simulink model "sim_WAM_PBRCDynamics"  (R2018b)
settings: Solver=FixedStepAuto  StartTime=0.0  StopTime=2  FixedStep=1e-3  RelTol=1e-3
values from neighbouring files (symbols this model uses):
  Cfcn = matlabFunction(Ctemp, 'vars', {q1, q2, q4, q1d, q2d, q4d})    [convertSymVarsTOfunctions.m]
  Ffcn = matlabFunction(Ftemp, 'vars', {q1d, q2d, q4d})    [convertSymVarsTOfunctions.m]
  Gfcn = matlabFunction(Gtemp, 'vars', {q1, q2, q4})    [convertSymVarsTOfunctions.m]
  handles =     [opt.mat]
  K = diag([10 30 10])    [MAIN_FINAL.m]    (also in PBMC_WAM.m = 10*diag([1 1 1]))
  Lambda = 5*eye(3)    [MAIN_FINAL.m]    (also in PBMC_WAM.m = 10*diag([1 1 1]))
  Mfcn = matlabFunction(Mtemp, 'vars', {q1, q2, q4})    [convertSymVarsTOfunctions.m]
  rho = 10    [MAIN_FINAL.m]
  TH0 = TH    [MAIN_FINAL.m]
  w = 2*pi/10    (= 0.628318530718)    [GetOptimalTrajectories.m]    (also in MAIN_FINAL.m = 1; MAIN_OptimalTrajectories.m; invDynWAM.m = 4; trajct1.mat)
  Yavfcn = matlabFunction(Yavtemp, 'vars', {q1, q2, q4, q1d, q2d, q4d, q1dd, q2dd, q4dd,                                                  v1, v2, v3, a1, a2, a3})    [convertSymVarsTOfunctions.m]
undefined symbols (not defined in the file or in its folder): getOptimal, PBRC_WAM, statederWAM
settings Model: Creator=Erivelton  LastModifiedBy=Erivelton

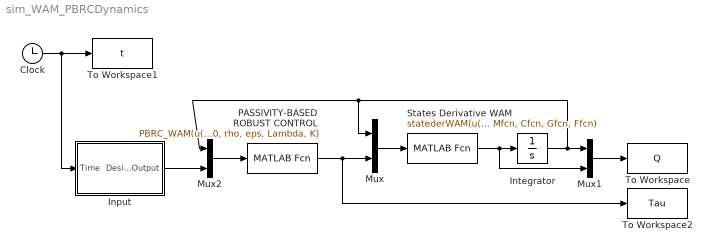
== system sim_WAM_PBRCDynamics ==
  Clock : Clock
  Input : Subsystem
  Integrator : Integrator  InitialCondition=handles.Q0
  Mux : Mux  Inputs=2
  Mux1 : Mux  Inputs=2
  Mux2 : Mux  Inputs=2
  PASSIVITY-BASED ROBUST CONTROL : MATLABFcn  MATLABFcn=PBRC_WAM(u(1:6), u(7:15), Yavfcn, TH0, rho, eps, Lambda, K)  OutputDimensions=3
  States Derivative WAM : MATLABFcn  MATLABFcn=statederWAM(u(1:6), u(7:9), Mfcn, Cfcn, Gfcn, Ffcn)  OutputDimensions=6
  To Workspace : ToWorkspace  VariableName=Q  SampleTime=-1
  To Workspace1 : ToWorkspace  VariableName=t  SampleTime=-1
  To Workspace2 : ToWorkspace  VariableName=Tau  SampleTime=-1
  wires:
  States Derivative WAM/1 -> Mux1/2, Integrator/1
  Mux/1 -> States Derivative WAM/1
  Integrator/1 -> Mux1/1, Mux/1, Mux2/1
  Clock/1 -> Input/1("Time "), To Workspace1/1
  Mux1/1 -> To Workspace/1
  PASSIVITY-BASED ROBUST CONTROL/1 -> To Workspace2/1, Mux/2
  Input/1(Desired Output) -> Mux2/2
  Mux2/1 -> PASSIVITY-BASED ROBUST CONTROL/1

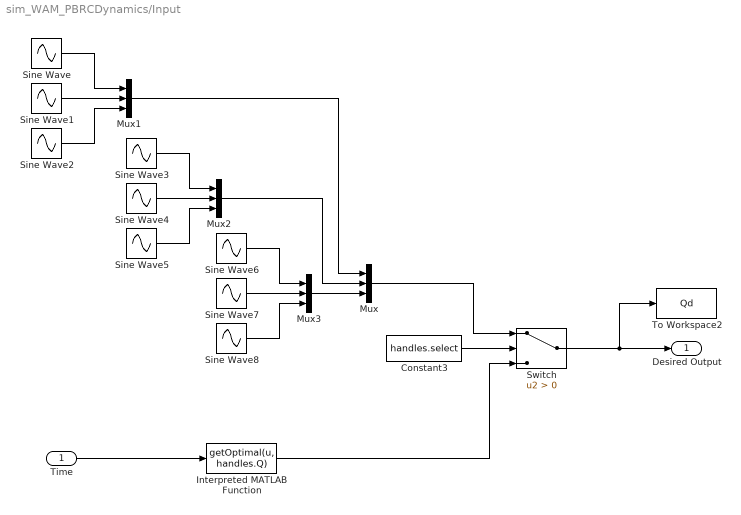
== system sim_WAM_PBRCDynamics/Input ==
  "Time " : Inport
  Constant3 : Constant  Value=handles.select
  Interpreted MATLAB Function : MATLABFcn  MATLABFcn=getOptimal(u, handles.Q)
  Mux{,1..3} (4 alike) : Mux  Inputs=3
  Sine Wave : Sin  Frequency=w  SampleTime=0
  Sine Wave1 : Sin  Amplitude=w  Frequency=w  Phase=pi/2  SampleTime=0
  Sine Wave2 : Sin  Amplitude=-w*w  Frequency=w  SampleTime=0
  Sine Wave3 : Sin  Bias=-.5  Frequency=w  SampleTime=0
  Sine Wave4 : Sin  Amplitude=w  Frequency=w  Phase=pi/2  SampleTime=0
  Sine Wave5 : Sin  Amplitude=-w*w  Frequency=w  SampleTime=0
  Sine Wave6 : Sin  Amplitude=.75  Frequency=w  SampleTime=0
  Sine Wave7 : Sin  Amplitude=.75*w  Frequency=w  Phase=pi/2  SampleTime=0
  Sine Wave8 : Sin  Amplitude=-.75*w*w  Frequency=w  SampleTime=0
  Switch : Switch  Criteria=u2 > Threshold
  To Workspace2 : ToWorkspace  VariableName=Qd  SampleTime=-1
  Desired Output : Outport
  wires:
  Mux/1 -> Switch/1
  Mux3/1 -> Mux/3
  Mux2/1 -> Mux/2
  Mux1/1 -> Mux/1
  Sine Wave/1 -> Mux1/1
  Sine Wave1/1 -> Mux1/2
  Sine Wave2/1 -> Mux1/3
  Sine Wave5/1 -> Mux2/3
  Sine Wave4/1 -> Mux2/2
  Sine Wave3/1 -> Mux2/1
  Sine Wave8/1 -> Mux3/3
  Sine Wave7/1 -> Mux3/2
  Sine Wave6/1 -> Mux3/1
  Constant3/1 -> Switch/2
  Switch/1 -> To Workspace2/1, Desired Output/1
  Interpreted MATLAB Function/1 -> Switch/3
  "Time "/1 -> Interpreted MATLAB Function/1
